simulink model "SIMULINK_Q36121333"  (R2023a)
settings: Solver=VariableStepAuto  StartTime=0.0  StopTime=0.002  FixedStep=2e-12  MaxStep=1e-7  RelTol=1e-3
undefined symbols (not defined in the file or in its folder): plecs
libraries: simulink x1
settings Model: Creator=stanl  LastModifiedBy=stanl
settings SolverCC: ConsecutiveZCsStepRelTol=10*1280*eps

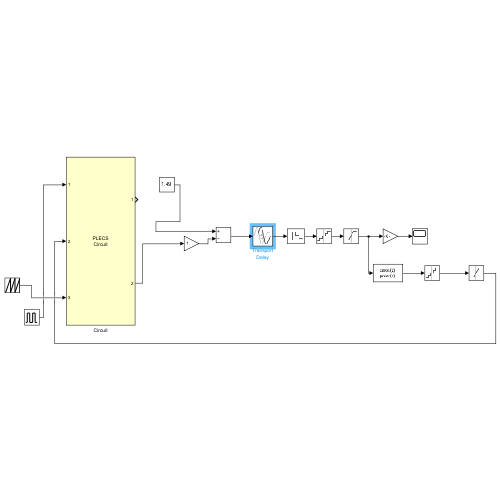
[thumbnail: Simulink's stored preview of the top-level diagram]
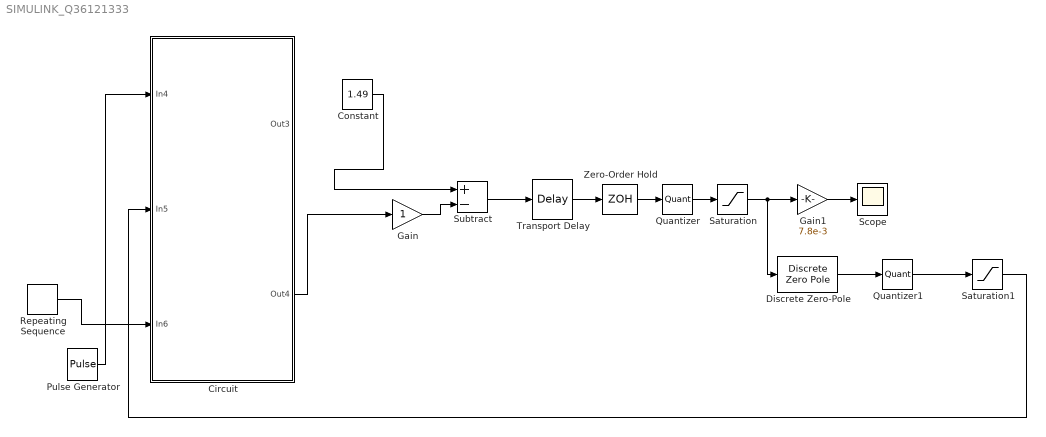
== system SIMULINK_Q36121333 ==
  Circuit : Subsystem  LoadFcn=plecs('sl', 200);  InitFcn=plecs('sl', 214);  StartFcn=plecs('sl', 208);  StopFcn=plecs('sl', 209);  mask(PlecsCircuit){PLECSData=<binary blob, 3736 chars, not shown>}
      mask prompts: PLECSData "PLECS Data (Do not delete or modify!)"
      mask init:
      | % PLACE CUSTOM INITIALIZATIONS ABOVE
      | % DO NOT REMOVE
      | plecs('sl', 215);
      | % DO NOT REMOVE
      settings: CopyFcn=plecs('sl', 203);  DeleteFcn=plecs('sl', 205);  UndoDeleteFcn=plecs('sl', 206);  PreSaveFcn=plecs('sl', 211);  PostSaveFcn=plecs('sl', 201);  NameChangeFcn=plecs('sl', 210);  DestroyFcn=plecs('sl', 207);  PreCopyFcn=plecs('sl', 216);  OpenFcn=plecs('sl', 202);  ErrorFcn=plerrorfcn
      mask Help: web(['file:///' fullfile(plecsdoc, 'creatingacircuit.html')])
      mask Display: disp('PLECS\nCircuit')
  Constant : Constant  Value=1.49
  Discrete Zero-Pole : DiscreteZeroPole  Zeros=[1 -0.9997]  Poles=[-0.6065 0.4671]  Gain=67.8937  SampleTime=-1
  Gain : Gain
  Gain1 : Gain  Gain=7.8e-3
  Pulse Generator : DiscretePulseGenerator  PulseType=Time based  Amplitude=5  Period=0.0005  PulseWidth=50  PhaseDelay=0.0002
  Quantizer : Quantizer  QuantizationInterval=15.625e-3
  Quantizer1 : Quantizer  QuantizationInterval=1/512
  Repeating Sequence : simulink/Sources/Repeating Sequence  rep_seq_t=[0 2e-6]  rep_seq_y=[0 3]
  Saturation : Saturate  UpperLimit=200.5e-3  LowerLimit=-10e-3
  Saturation1 : Saturate  UpperLimit=0.95  LowerLimit=0.05
  Scope : Scope
  Subtract : Sum  Inputs=+-
  Transport Delay : TransportDelay  DelayTime=4.95e-7  InitialOutput=1.5
  Zero-Order Hold : ZeroOrderHold  SampleTime=1e-6
  wires:
  Pulse Generator/1 -> Circuit/1(In4)
  Repeating Sequence/1 -> Circuit/3(In6)
  Circuit/2(Out4) -> Gain/1
  Gain/1 -> Subtract/2
  Constant/1 -> Subtract/1
  Subtract/1 -> Transport Delay/1
  Transport Delay/1 -> Zero-Order Hold/1
  Zero-Order Hold/1 -> Quantizer/1
  Quantizer/1 -> Saturation/1
  Saturation/1 -> Discrete Zero-Pole/1, Gain1/1
  Gain1/1 -> Scope/1
  Discrete Zero-Pole/1 -> Quantizer1/1
  Quantizer1/1 -> Saturation1/1
  Saturation1/1 -> Circuit/2(In5)

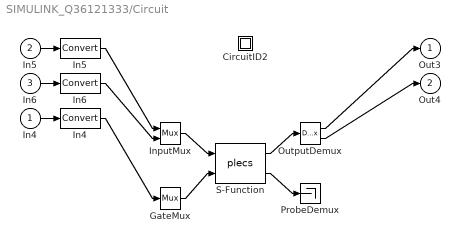
== system SIMULINK_Q36121333/Circuit ==
  In4 : Inport  PortDimensions=1
  In5 : Inport  Port=2  PortDimensions=1
  In6 : Inport  Port=3  PortDimensions=1
  " CircuitID2 " : Subsystem
  " GateMux " : Mux  Inputs=[ 1 ]
  " In4 " : DataTypeConversion
  " In5 " : DataTypeConversion
  " In6 " : DataTypeConversion
  " InputMux " : Mux  Inputs=[ 1 1 ]
  " OutputDemux " : Demux  Outputs=[ 1 1 ]
  " ProbeDemux " : Terminator
  " S-Function " : S-Function  FunctionName=plecs  SFunctionDeploymentMode=off  EnableBusSupport=off
  Out3 : Outport  PortDimensions=1
  Out4 : Outport  Port=2  PortDimensions=1
  wires:
  " InputMux "/1 -> " S-Function "/1
  " GateMux "/1 -> " S-Function "/2
  " S-Function "/1 -> " OutputDemux "/1
  " S-Function "/2 -> " ProbeDemux "/1
  In5/1 -> " In5 "/1
  " In5 "/1 -> " InputMux "/1
  In6/1 -> " In6 "/1
  " In6 "/1 -> " InputMux "/2
  In4/1 -> " In4 "/1
  " In4 "/1 -> " GateMux "/1
  " OutputDemux "/1 -> Out3/1
  " OutputDemux "/2 -> Out4/1

== system SIMULINK_Q36121333/Circuit/ CircuitID2  ==
